simulink model "VORmodel"  (R2025b)
settings: Solver=VariableStepAuto  StartTime=0.0  StopTime=600  RelTol=1e-3
values from neighbouring files (symbols this model uses):
  A_red = SS_lat_lo.A(id_x, id_x)    [VORReducedModel.m]
  B_red = SS_lat_lo.A(id_x, id_u)    [VORReducedModel.m]
  C_red = SS_lat_lo.C([6,5,4], id_x)    [VORReducedModel.m]
  D_red = zeros(3,2)    [VORReducedModel.m]
  velocity = input('Enter the velocity for the simulation (ft/s):  ')    [FindF16Dynamics.m]
libraries: simulink_extras x3
settings Model: Creator=pprochacki  LastModifiedBy=pprochacki

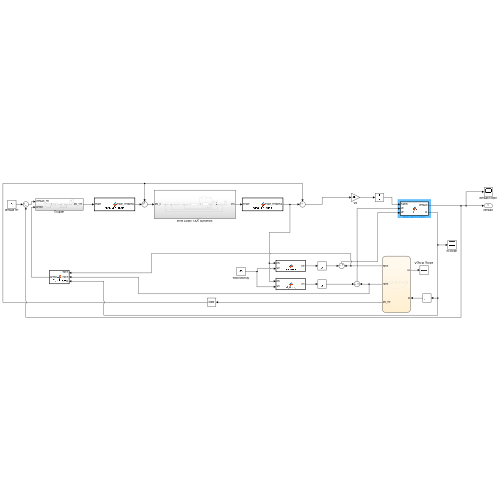
[thumbnail: Simulink's stored preview of the top-level diagram]
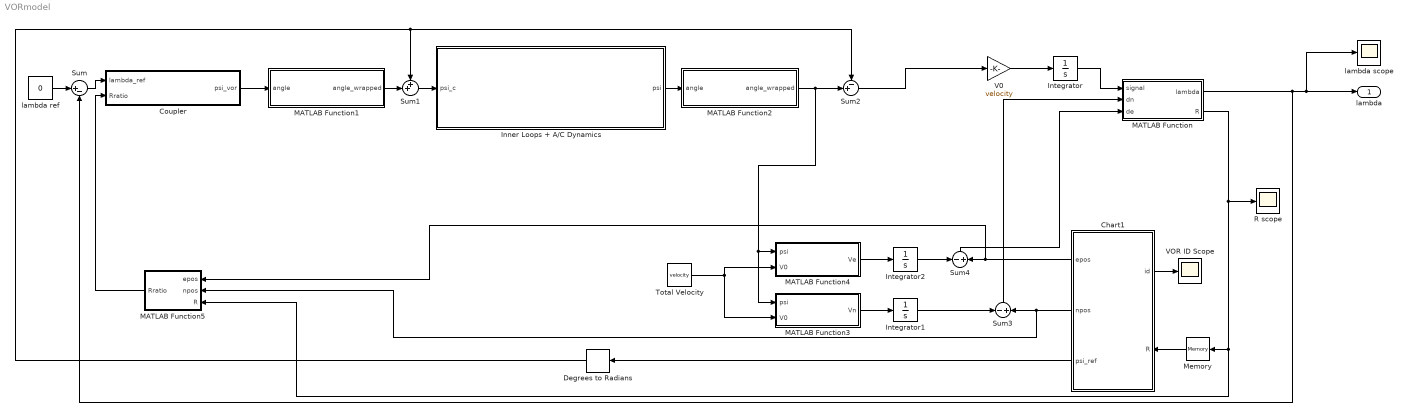
== system VORmodel ==
  Chart1 : Stateflow chart  TreatAsAtomicUnit=on
      settings: PortSchema="{\"entries\":[{\"content\":{\"sides\":[{\"content\":{\"connectorIds\":[\"Out1\",\"In1\"]},\"type\":\"ConnectorPlacement.EquallySpacedRectSide\",\"uuid\":\"33511b5d-7d68-47cc-afe3-9b99f8d571de\"},{\"content\":{\"connectorIds\":[\"Out3\",\"Out2\",\"Out4\"],\"side\":\"RIGHT\"},\"type\":\"ConnectorPlacement.EquallySpacedRectSide\",\"uuid\":\"9fd47d51-d0cf-4061-b21e-ccacd4b92614\"},{\"content\":{\"side\":\"TOP\"},\"type\":\"ConnectorPlacement.EquallySpacedRectSide\",\"uuid\":\"73041c2e-dff9-4c9c-8efb-53cb0456c1ae\"}]},\"type\":\"ConnectorPlacement.EquallySpacedConnector\",\"uuid\":\"f315a1bd-26df-42d9-b94f-94c36dc396f8\"}],\"packageUris\":[\"http://schema.mathworks.com/mf0/Connector/R2020b\"],\"version\":\"1.0\"}"
  Coupler : Subsystem
  Degrees to Radians : simulink_extras/Transformations/Degrees to Radians
  Inner Loops + A/C Dynamics : Subsystem
  Integrator : Integrator
  Integrator1 : Integrator
  Integrator2 : Integrator
  MATLAB Function : MATLAB Function  TreatAsAtomicUnit=on
  MATLAB Function1 : MATLAB Function  TreatAsAtomicUnit=on
  MATLAB Function2 : MATLAB Function  TreatAsAtomicUnit=on
  MATLAB Function3 : MATLAB Function  TreatAsAtomicUnit=on
  MATLAB Function4 : MATLAB Function  TreatAsAtomicUnit=on
  MATLAB Function5 : MATLAB Function  TreatAsAtomicUnit=on
  Memory : Memory
  R scope : Scope
      settings: ActiveDisplayYMinimum=-19286.771145697858  ActiveDisplayYMaximum=310336.65252777375  DataLoggingVariableName=ScopeData7
  Sum : Sum  Inputs=|+-
  Sum1 : Sum  Inputs=++|
  Sum2 : Sum  Inputs=-+|
  Sum3 : Sum  Inputs=-|+
  Sum4 : Sum  Inputs=-|+
  Total Velocity : Constant  Value=velocity
  V0 : Gain  Gain=velocity
  VOR ID Scope : Scope
      settings: ActiveDisplayYMinimum=0.9  ActiveDisplayYMaximum=1.1  DataLoggingVariableName=ScopeData5
  lambda ref : Constant  Value=0
  lambda scope : Scope
      settings: ActiveDisplayYMinimum=-4.5671508576563937  ActiveDisplayYMaximum=4.3012604666646492  DataLoggingVariableName=ScopeData6
  lambda : Outport
  wires:
  Sum/1 -> Coupler/1(lambda_ref)
  Coupler/1(psi_vor) -> MATLAB Function1/1(angle)
  Sum1/1 -> Inner Loops + A/C Dynamics/1(psi_c)
  Inner Loops + A/C Dynamics/1(psi) -> MATLAB Function2/1(angle)
  V0/1 -> Integrator/1
  lambda ref/1 -> Sum/1
  Memory/1 -> Chart1/1(R)
  Integrator/1 -> MATLAB Function/1(signal)
  MATLAB Function/1(lambda) -> lambda scope/1, lambda/1, Sum/2
  MATLAB Function/2(R) -> R scope/1, MATLAB Function5/3(R), Memory/1
  Chart1/1(id) -> VOR ID Scope/1
  MATLAB Function3/1(Vn) -> Integrator1/1
  MATLAB Function4/1(Ve) -> Integrator2/1
  Integrator1/1 -> Sum3/1
  Chart1/3(epos) -> MATLAB Function5/1(epos), Sum4/2
  Integrator2/1 -> Sum4/1
  Chart1/2(npos) -> MATLAB Function5/2(npos), Sum3/2
  Sum4/1 -> MATLAB Function/3(de)
  Sum3/1 -> MATLAB Function/2(dn)
  Chart1/4(psi_ref) -> Degrees to Radians/1
  Degrees to Radians/1 -> Sum1/1, Sum2/1
  MATLAB Function1/1(angle_wrapped) -> Sum1/2
  Sum2/1 -> V0/1
  Total Velocity/1 -> MATLAB Function3/2(V0), MATLAB Function4/2(V0)
  MATLAB Function5/1(Rratio) -> Coupler/2(Rratio)
  MATLAB Function2/1(angle_wrapped) -> MATLAB Function3/1(psi), MATLAB Function4/1(psi), Sum2/2

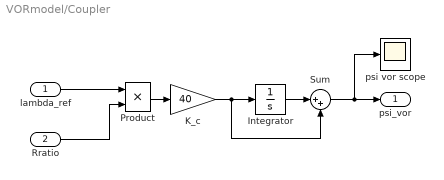
== system VORmodel/Coupler ==
  lambda_ref : Inport
  Rratio : Inport  Port=2
  Integrator : Integrator
  K_c : Gain  Gain=40
  Product : Product
  Sum : Sum  Inputs=|++
  psi vor scope : Scope
      settings: ActiveDisplayYMinimum=-10604.634260735544  ActiveDisplayYMaximum=95441.708346619911  DataLoggingVariableName=ScopeData4
  psi_vor : Outport
  wires:
  Integrator/1 -> Sum/1
  Sum/1 -> psi vor scope/1, psi_vor/1
  lambda_ref/1 -> Product/1
  K_c/1 -> Sum/2, Integrator/1
  Rratio/1 -> Product/2
  Product/1 -> K_c/1

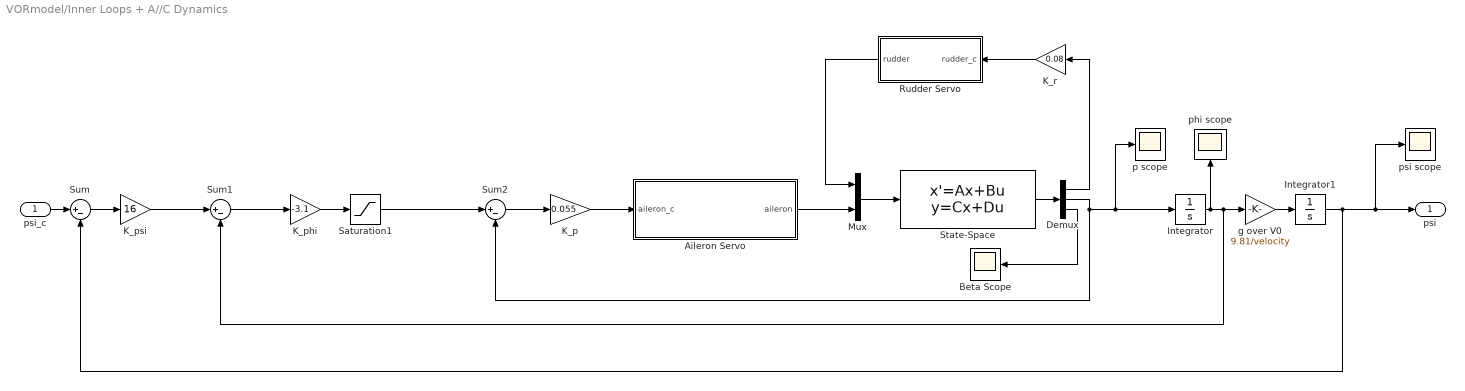
== system VORmodel/Inner Loops + A//C Dynamics ==
  psi_c : Inport
  Aileron Servo : Subsystem
  Beta Scope : Scope
      settings: ActiveDisplayYMinimum=-0.069952877696829938  ActiveDisplayYMaximum=0.073344065412398241
  Demux : Demux  Outputs=3
  Integrator : Integrator
  Integrator1 : Integrator
  K_p : Gain  Gain=0.055
  K_phi : Gain  Gain=-3.1
  K_psi : Gain  Gain=16
  K_r : Gain  Gain=0.08
  Mux : Mux  Inputs=2
  Rudder Servo : Subsystem
  Saturation1 : Saturate  UpperLimit=60*pi/180  LowerLimit=-60*pi/180
  State-Space : StateSpace  A=A_red  B=B_red  C=C_red  D=D_red  InitialCondition=0
  Sum : Sum  Inputs=|+-
  Sum1 : Sum  Inputs=|+-
  Sum2 : Sum  Inputs=|+-
  g over V0 : Gain  Gain=9.81/velocity
  p scope : Scope
      settings: ActiveDisplayYMinimum=-0.47648345709462181  ActiveDisplayYMaximum=0.39014127584639091  DataLoggingVariableName=ScopeData2
  phi scope : Scope
      settings: ActiveDisplayYMinimum=-0.63211616387848069  ActiveDisplayYMaximum=1.5690456204817835  DataLoggingVariableName=ScopeData3
  psi scope : Scope
      settings: ActiveDisplayYMinimum=-6.73006939362087  ActiveDisplayYMaximum=3.6241970984012992
  psi : Outport
  wires:
  Sum1/1 -> K_phi/1
  Sum2/1 -> K_p/1
  g over V0/1 -> Integrator1/1
  Integrator1/1 -> Sum/2, psi scope/1, psi/1
  Integrator/1 -> g over V0/1, Sum1/2, phi scope/1
  Aileron Servo/1(aileron) -> Mux/2
  Rudder Servo/1(rudder) -> Mux/1
  Mux/1 -> State-Space/1
  K_r/1 -> Rudder Servo/1(rudder_c)
  State-Space/1 -> Demux/1
  Demux/2 -> p scope/1, Integrator/1, Sum2/2
  Demux/1 -> K_r/1
  Demux/3 -> Beta Scope/1
  K_p/1 -> Aileron Servo/1(aileron_c)
  K_phi/1 -> Saturation1/1
  Sum/1 -> K_psi/1
  Saturation1/1 -> Sum2/1
  K_psi/1 -> Sum1/1
  psi_c/1 -> Sum/1

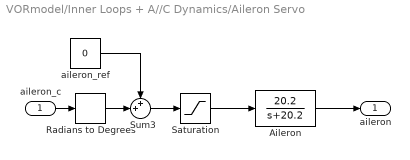
== system VORmodel/Inner Loops + A//C Dynamics/Aileron Servo ==
  aileron_c : Inport
  Aileron : TransferFcn  Numerator=[20.2]  Denominator=[1 20.2]
  Radians to Degrees : simulink_extras/Transformations/Radians to Degrees
  Saturation : Saturate  UpperLimit=21.5  LowerLimit=-21.5
  Sum3 : Sum  Inputs=++|
  aileron_ref : Constant  Value=0
  aileron : Outport
  wires:
  aileron_ref/1 -> Sum3/1
  Saturation/1 -> Aileron/1
  Aileron/1 -> aileron/1
  aileron_c/1 -> Radians to Degrees/1
  Radians to Degrees/1 -> Sum3/2
  Sum3/1 -> Saturation/1

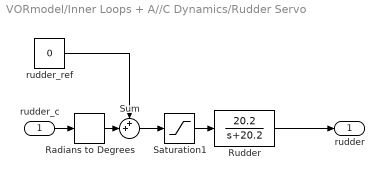
== system VORmodel/Inner Loops + A//C Dynamics/Rudder Servo ==
  rudder_c : Inport
  Radians to Degrees : simulink_extras/Transformations/Radians to Degrees
  Rudder : TransferFcn  Numerator=[20.2]  Denominator=[1 20.2]
  Saturation1 : Saturate  UpperLimit=30  LowerLimit=-30
  Sum : Sum  Inputs=++|
  rudder_ref : Constant  Value=0
  rudder : Outport
  wires:
  rudder_c/1 -> Radians to Degrees/1
  Rudder/1 -> rudder/1
  rudder_ref/1 -> Sum/1
  Saturation1/1 -> Rudder/1
  Sum/1 -> Saturation1/1
  Radians to Degrees/1 -> Sum/2

== stateflow chart VORmodel/Chart1 ==
  settings: updateMethod=DISCRETE  sampleTime=0.1
  state beacon1
    id=1;
    npos=15000;
    epos=15000;
    psi_ref=45;
  state beacon2
    id=2;
    npos=0;
    epos=30000;
    psi_ref=135;
  state beacon3
    id=3;
    npos=-15000;
    epos=30000;
    psi_ref=180;
  state beacon4
    id=4;
    npos=-30000;
    epos=45000;
    psi_ref=135;
  state beacon5
    id=5;
    npos=0;
    epos=0;
    psi_ref=0;
  (default) -> beacon1
  beacon2 -> beacon3 : [R<5000]
  beacon3 -> beacon4 : [R<5000]
  beacon1 -> beacon2 : [R<5000]
  beacon4 -> beacon5 : [R<5000]
  beacon5 -> beacon1 : [R<5000]
  data: R input; id output; npos output; epos output; psi_ref output

== matlab function VORmodel/MATLAB Function ==
  data: lambda output; signal input; dn input; R output; de input
function [lambda, R]= R(signal, dn, de)

R = sqrt(dn^2 + de^2);
lambda = signal/R ;

== matlab function VORmodel/MATLAB Function1 ==
  data: angle input; angle_wrapped output
function angle_wrapped = constrain_angle(angle)
    angle_wrapped = wrapToPi(angle);
end

== matlab function VORmodel/MATLAB Function2 ==
  data: angle input; angle_wrapped output
function angle_wrapped = constrain_angle(angle)
    angle_wrapped = wrapToPi(angle);
end

== matlab function VORmodel/MATLAB Function3 ==
  data: psi input; Vn output; V0 input
function Vn = calcVnorth(psi, V0)
Vn = V0 * cos(psi);

== matlab function VORmodel/MATLAB Function4 ==
  data: psi input; Ve output; V0 input
function Ve = calcVeast(psi, V0)
Ve = V0 * sin(psi);

== matlab function VORmodel/MATLAB Function5 ==
  data: epos input; npos input; Rratio output; R input
function Rratio = CalcRratio(epos, npos, R)

R0 = sqrt(npos^2+epos^2);
Rratio = R/R0;
